simulink model "Laengsdynamikmodell"  (R2018b)
settings: Solver=ode4  StartTime=0.0  StopTime=10.0  FixedStep=0.001  RelTol=1e-3
model workspace (MAT data in the model file):
  controllerActive = 0
  g = 9.81
  hs = 0.5
  l = 2.8
  lv = 1.344
  rBreakpoints = [0 0.25 1]
  rTableData = [0 1 1]
  reifenX = [0 0.25 1]
  reifenY = [0 1 1]
  useController = 0
  v0 = 22.2222222222
  zBreakpoints = [0.01 0.02 0.03 0.04 0.05 0.06 0.07 0.08 0.09 0.1 0.11 0.12 ... (561 elements, 1x561)]
  zTableData = [-2.912 -2.902 -2.892 -2.882 -2.872 -2.862 -2.852 -2.842 -2.832 -2.822 -2.812 -2.802 ... (561 elements, 1x561)]
  z_time = [0.01 0.02 0.03 0.04 0.05 0.06 0.07 0.08 0.09 0.1 0.11 0.12 ... (561 elements, 1x561)]
  z_vals = [-2.912 -2.902 -2.892 -2.882 -2.872 -2.862 -2.852 -2.842 -2.832 -2.822 -2.812 -2.802 ... (561 elements, 1x561)]
  zh_z = 1
  zv_z = 1
undefined symbols (not defined in the file or in its folder): z_values
settings Model: Creator=gregoryseibert  LastModifiedBy=gregoryseibert

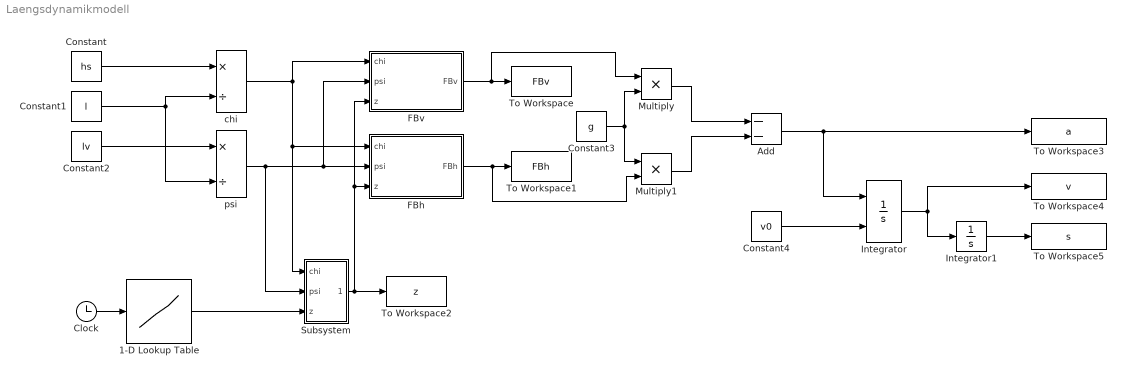
== system Laengsdynamikmodell ==
  1-D Lookup Table : Lookup_n-D  NumberOfTableDimensions=1  BreakpointsForDimension1=z_time  Table=z_values  InternalRulePriority=Speed  RndMeth=Simplest  InputSameDT=on
  Add : Sum  Inputs=--
  Clock : Clock
  Constant : Constant  Value=hs
  Constant1 : Constant  Value=l
  Constant2 : Constant  Value=lv
  Constant3 : Constant  Value=g
  Constant4 : Constant  Value=v0
  FBh : Subsystem
  FBv : Subsystem
  Integrator : Integrator  InitialConditionSource=external  LimitOutput=on  LowerSaturationLimit=0
  Integrator1 : Integrator
  Multiply : Product
  Multiply1 : Product
  Subsystem : Subsystem
  To Workspace : ToWorkspace  VariableName=FBv  SampleTime=-1
      settings: Save2DSignal=2-D array (concatenate along first dimension)
  To Workspace1 : ToWorkspace  VariableName=FBh  SampleTime=-1
      settings: Save2DSignal=2-D array (concatenate along first dimension)
  To Workspace2 : ToWorkspace  VariableName=z  SampleTime=-1
      settings: Save2DSignal=2-D array (concatenate along first dimension)
  To Workspace3 : ToWorkspace  VariableName=a  SaveFormat=Timeseries  SampleTime=-1
  To Workspace4 : ToWorkspace  VariableName=v  SaveFormat=Timeseries  SampleTime=-1
  To Workspace5 : ToWorkspace  VariableName=s  SaveFormat=Timeseries  SampleTime=-1
  chi : Product  Inputs=*/
  psi : Product  Inputs=*/
  wires:
  Constant/1 -> chi/1
  Constant1/1 -> chi/2, psi/2
  Constant2/1 -> psi/1
  chi/1 -> Subsystem/1(chi), FBh/1(chi), FBv/1(chi)
  psi/1 -> Subsystem/2(psi), FBv/2(psi), FBh/2(psi)
  Clock/1 -> 1-D Lookup Table/1
  FBh/1(FBh) -> Multiply1/2, To Workspace1/1
  FBv/1(FBv) -> Multiply/1, To Workspace/1
  Subsystem/1(zOut) -> To Workspace2/1, FBv/3(z), FBh/3(z)
  1-D Lookup Table/1 -> Subsystem/3(z)
  Multiply/1 -> Add/1
  Constant4/1 -> Integrator/2
  Add/1 -> Integrator/1, To Workspace3/1
  Integrator1/1 -> To Workspace5/1
  Multiply1/1 -> Add/2
  Integrator/1 -> Integrator1/1, To Workspace4/1
  Constant3/1 -> Multiply1/1, Multiply/2

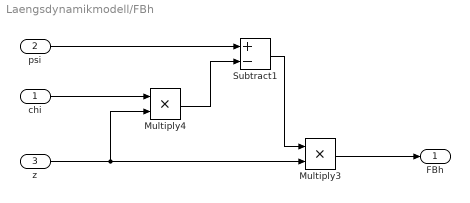
== system Laengsdynamikmodell/FBh ==
  chi : Inport
  psi : Inport  Port=2
  z : Inport  Port=3
  Multiply3 : Product
  Multiply4 : Product
  Subtract1 : Sum  Inputs=+-
  FBh : Outport
  wires:
  chi/1 -> Multiply4/1
  Multiply3/1 -> FBh/1
  psi/1 -> Subtract1/1
  Subtract1/1 -> Multiply3/1
  Multiply4/1 -> Subtract1/2
  z/1 -> Multiply4/2, Multiply3/2

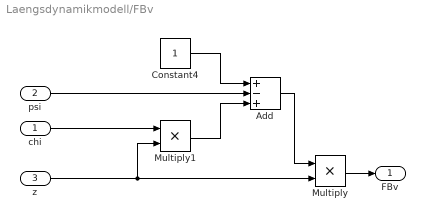
== system Laengsdynamikmodell/FBv ==
  chi : Inport
  psi : Inport  Port=2
  z : Inport  Port=3
  Add : Sum  Inputs=+-+
  Constant4 : Constant
  Multiply : Product
  Multiply1 : Product
  FBv : Outport
  wires:
  psi/1 -> Add/2
  Add/1 -> Multiply/1
  Multiply1/1 -> Add/3
  Constant4/1 -> Add/1
  chi/1 -> Multiply1/1
  Multiply/1 -> FBv/1
  z/1 -> Multiply1/2, Multiply/2

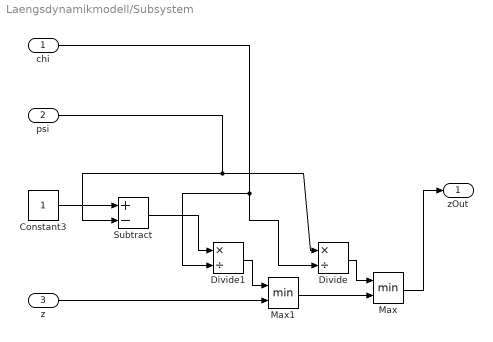
== system Laengsdynamikmodell/Subsystem ==
  chi : Inport
  psi : Inport  Port=2
  z : Inport  Port=3
  Constant3 : Constant
  Divide : Product  Inputs=*/
  Divide1 : Product  Inputs=*/
  Max : MinMax  Inputs=2
  Max1 : MinMax  Inputs=2
  Subtract : Sum  Inputs=+-
  zOut : Outport
  wires:
  Max/1 -> zOut/1
  z/1 -> Max1/2
  chi/1 -> Divide/2, Divide1/2
  Divide1/1 -> Max1/1
  Constant3/1 -> Subtract/1
  Divide/1 -> Max/1
  Max1/1 -> Max/2
  psi/1 -> Divide/1, Subtract/2
  Subtract/1 -> Divide1/1
